simulink model "hexa_CAD_FxTDiff_ANSFT"  (R2023a)
settings: Solver=ode4  StartTime=0.0  StopTime=60  FixedStep=0.01  RelTol=1e-3
model workspace (MAT data in the model file):
  hover_2m = [0 0 2 0 0 0 0 0 2 0 0 0 ... (36 elements, 6x6)]
  square = [0 0 2.5 0 0 0 0 0 2.5 0 0 0 ... (36 elements, 6x6)]
  tf : Simulink.Parameter (value not decoded)
  tray0 = [0 0 0 0 0 0 0 0 5 0 0 0 ... (36 elements, 6x6)]
  tray1 = [0 0 0 0 0 0 0 0 5 0 0 0 ... (36 elements, 6x6)]
  tray2 = [0 0 0 0 0 0 2 0 5 0 0 0 ... (36 elements, 6x6)]
  tray3 = [0 0 0 0 0 0 2 0 5 0 0 0 ... (36 elements, 6x6)]
  tray4 = [0 0 0 0 0 0 2 0 5 0.15 0 0 ... (36 elements, 6x6)]
  tray5 = [0 0 0 0 0 0 0 0 5 0.15 0 0 ... (36 elements, 6x6)]
  tray_roll = [0 0 0 0.15 0 0 0 0 0 0.15 0 0 ... (36 elements, 6x6)]
  tray_yaw = [0 0 0 0 0 0 0 0 5 0 0 0 ... (36 elements, 6x6)]
undefined symbols (not defined in the file or in its folder): F, Light, MIL, smiData, X, Y, Z
libraries: sm_lib x230, nesl_utility x28, dspsrcs4 x6, simulink x3, sharedtransform x2, robotcorelib x1, aerolibwind2 x1, SignalEditorBlockLib x1
(part 6 of 6)

== system hexa_CAD_FxTDiff_ANSFT/6DoF_Dynamics/Hexa_Simsape/Raspberry_Pi_4_Model_B_STEP_1_RIGID/x2X_USB2_0_PORTS_RPi4ModelB_STEP_1_RIGID ==
  ReferenceFrame : sm_lib/Frames and Transforms/Reference Frame
  Solid : sm_lib/Body Elements/File Solid  ExtGeomFileName=2X USB2.0 PORTS- RPi4ModelB.STEP_Predeterminado_sldprt.STEP  UnitType=FromFile  ExtGeomFileUnits=m  StepReaderType=HEX  ExportConvexHullGeometry=off  InertiaType=Custom  Mass=smiData.Solid(25).mass  MassUnits=kg  CenterOfMass=smiData.Solid(25).CoM  CenterOfMassUnits=mm  MomentsOfInertia=smiData.Solid(25).MoI  MomentsOfInertiaUnits=kg*mm^2  ProductsOfInertia=smiData.Solid(25).PoI  ProductsOfInertiaUnits=kg*mm^2  BasedOnType=DensityFromFile  Density=1000  DensityUnits=kg/m^3  DoExposeReferenceFrame=on  SerializedFrames=<Frames/>  GraphicType=FromGeometry  MarkerShape=Sphere  MarkerSize=10  GraphicVisPropType=SimpleVisualProperties  GraphicDiffuseColor=smiData.Solid(25).color  GraphicSpecularColor=[0.5 0.5 0.5 1.0]  GraphicAmbientColor=[0.15 0.15 0.15 1.0]  GraphicEmissiveColor=[0.0 0.0 0.0 1.0]  GraphicShininess=75  GraphicOpacity=smiData.Solid(25).opacity
  F : PMIOPort  Side=Left
  connections:
  Solid/RConn1 -- ReferenceFrame/RConn1 -- F/RConn1

== system hexa_CAD_FxTDiff_ANSFT/6DoF_Dynamics/Hexa_Simsape/Raspberry_Pi_4_Model_B_STEP_1_RIGID/x2X_USB3_0_PORTS_RPi4ModelB_STEP_1_RIGID ==
  ReferenceFrame : sm_lib/Frames and Transforms/Reference Frame
  Solid : sm_lib/Body Elements/File Solid  ExtGeomFileName=2X USB3.0 PORTS- RPi4ModelB.STEP_Predeterminado_sldprt.STEP  UnitType=FromFile  ExtGeomFileUnits=m  StepReaderType=HEX  ExportConvexHullGeometry=off  InertiaType=Custom  Mass=smiData.Solid(11).mass  MassUnits=kg  CenterOfMass=smiData.Solid(11).CoM  CenterOfMassUnits=mm  MomentsOfInertia=smiData.Solid(11).MoI  MomentsOfInertiaUnits=kg*mm^2  ProductsOfInertia=smiData.Solid(11).PoI  ProductsOfInertiaUnits=kg*mm^2  BasedOnType=DensityFromFile  Density=1000  DensityUnits=kg/m^3  DoExposeReferenceFrame=on  SerializedFrames=<Frames/>  GraphicType=FromGeometry  MarkerShape=Sphere  MarkerSize=10  GraphicVisPropType=SimpleVisualProperties  GraphicDiffuseColor=smiData.Solid(11).color  GraphicSpecularColor=[0.5 0.5 0.5 1.0]  GraphicAmbientColor=[0.15 0.15 0.15 1.0]  GraphicEmissiveColor=[0.0 0.0 0.0 1.0]  GraphicShininess=75  GraphicOpacity=smiData.Solid(11).opacity
  F : PMIOPort  Side=Left
  connections:
  Solid/RConn1 -- ReferenceFrame/RConn1 -- F/RConn1

== system hexa_CAD_FxTDiff_ANSFT/6DoF_Dynamics/Hexa_Simsape/Raspberry_Pi_4_Model_B_STEP_1_RIGID/x2_54_mm_DUPONT_MALE_PIN_HEADER_IO_2X20_RPi4ModelB_STEP_1_RIGID ==
  ReferenceFrame : sm_lib/Frames and Transforms/Reference Frame
  Solid : sm_lib/Body Elements/File Solid  ExtGeomFileName=2.54 mm DUPONT MALE PIN HEADER- IO- 2X20- RPi4ModelB.STEP_Predeterminado_sldprt.STEP  UnitType=FromFile  ExtGeomFileUnits=m  StepReaderType=HEX  ExportConvexHullGeometry=off  InertiaType=Custom  Mass=smiData.Solid(21).mass  MassUnits=kg  CenterOfMass=smiData.Solid(21).CoM  CenterOfMassUnits=mm  MomentsOfInertia=smiData.Solid(21).MoI  MomentsOfInertiaUnits=kg*mm^2  ProductsOfInertia=smiData.Solid(21).PoI  ProductsOfInertiaUnits=kg*mm^2  BasedOnType=DensityFromFile  Density=1000  DensityUnits=kg/m^3  DoExposeReferenceFrame=on  SerializedFrames=<Frames/>  GraphicType=FromGeometry  MarkerShape=Sphere  MarkerSize=10  GraphicVisPropType=SimpleVisualProperties  GraphicDiffuseColor=smiData.Solid(21).color  GraphicSpecularColor=[0.5 0.5 0.5 1.0]  GraphicAmbientColor=[0.15 0.15 0.15 1.0]  GraphicEmissiveColor=[0.0 0.0 0.0 1.0]  GraphicShininess=75  GraphicOpacity=smiData.Solid(21).opacity
  F : PMIOPort  Side=Left
  connections:
  Solid/RConn1 -- ReferenceFrame/RConn1 -- F/RConn1

== system hexa_CAD_FxTDiff_ANSFT/6DoF_Dynamics/Hexa_Simsape/Raspberry_Pi_4_Model_B_STEP_1_RIGID/x2_54_mm_DUPONT_MALE_PIN_HEADER_POE_2X2_RPi4ModelB_STEP_1_RIGID ==
  ReferenceFrame : sm_lib/Frames and Transforms/Reference Frame
  Solid : sm_lib/Body Elements/File Solid  ExtGeomFileName=2.54 mm DUPONT MALE PIN HEADER- POE- 2X2- RPi4ModelB.STEP_Predeterminado_sldprt.STEP  UnitType=FromFile  ExtGeomFileUnits=m  StepReaderType=HEX  ExportConvexHullGeometry=off  InertiaType=Custom  Mass=smiData.Solid(20).mass  MassUnits=kg  CenterOfMass=smiData.Solid(20).CoM  CenterOfMassUnits=mm  MomentsOfInertia=smiData.Solid(20).MoI  MomentsOfInertiaUnits=kg*mm^2  ProductsOfInertia=smiData.Solid(20).PoI  ProductsOfInertiaUnits=kg*mm^2  BasedOnType=DensityFromFile  Density=1000  DensityUnits=kg/m^3  DoExposeReferenceFrame=on  SerializedFrames=<Frames/>  GraphicType=FromGeometry  MarkerShape=Sphere  MarkerSize=10  GraphicVisPropType=SimpleVisualProperties  GraphicDiffuseColor=smiData.Solid(20).color  GraphicSpecularColor=[0.5 0.5 0.5 1.0]  GraphicAmbientColor=[0.15 0.15 0.15 1.0]  GraphicEmissiveColor=[0.0 0.0 0.0 1.0]  GraphicShininess=75  GraphicOpacity=smiData.Solid(20).opacity
  F : PMIOPort  Side=Left
  connections:
  Solid/RConn1 -- ReferenceFrame/RConn1 -- F/RConn1

== system hexa_CAD_FxTDiff_ANSFT/6DoF_Dynamics/Hexa_Simsape/Raspberry_Pi_4_Model_B_STEP_1_RIGID/x91D77_D9WHV_778K_4_GB_LPDDR4_SDRAM_RPi4ModelB_STEP_1_RIGID ==
  ReferenceFrame : sm_lib/Frames and Transforms/Reference Frame
  Solid : sm_lib/Body Elements/File Solid  ExtGeomFileName=91D77 D9WHV 778K- 4 GB LPDDR4 SDRAM- RPi4ModelB.STEP_Predeterminado_sldprt.STEP  UnitType=FromFile  ExtGeomFileUnits=m  StepReaderType=HEX  ExportConvexHullGeometry=off  InertiaType=Custom  Mass=smiData.Solid(13).mass  MassUnits=kg  CenterOfMass=smiData.Solid(13).CoM  CenterOfMassUnits=mm  MomentsOfInertia=smiData.Solid(13).MoI  MomentsOfInertiaUnits=kg*mm^2  ProductsOfInertia=smiData.Solid(13).PoI  ProductsOfInertiaUnits=kg*mm^2  BasedOnType=DensityFromFile  Density=1000  DensityUnits=kg/m^3  DoExposeReferenceFrame=on  SerializedFrames=<Frames/>  GraphicType=FromGeometry  MarkerShape=Sphere  MarkerSize=10  GraphicVisPropType=SimpleVisualProperties  GraphicDiffuseColor=smiData.Solid(13).color  GraphicSpecularColor=[0.5 0.5 0.5 1.0]  GraphicAmbientColor=[0.15 0.15 0.15 1.0]  GraphicEmissiveColor=[0.0 0.0 0.0 1.0]  GraphicShininess=75  GraphicOpacity=smiData.Solid(13).opacity
  F : PMIOPort  Side=Left
  connections:
  Solid/RConn1 -- ReferenceFrame/RConn1 -- F/RConn1

== matlab function hexa_CAD_FxTDiff_ANSFT/Trajectory/Helicoidal Trajectory ==
  data: time input; pose_d output; pose_d_dot output; pose_d_ddot output
function [pose_d, pose_d_dot, pose_d_ddot]= fcn(time)

% pos_z = time / 12;
f = 0.15;
arg = f * (time - 5);
r = 2;

% hover for 5 s | include inclination in roll
% 5 metros al menos

if (time < 5)
    pos_x = 0;
    pos_y = 0;
    roll = 0;
    pos_z = 0.4 * time;
    yaw = 0;
else
    pos_x = -r + r * cos (arg);
    pos_y = r * sin (arg);
    pos_z = 2;
    roll = 0.15;
    yaw = (time - 5) * 2 * pi / 180; 
end

% roll = 0;
% yaw = time * 0;

pose_d = [pos_x;
          pos_y;
          pos_z;
          roll;
          0;
          yaw*0];

% pos_z_dot = 1 / 12;

% hover for 5 s
if (time < 5)
    pos_x_dot = 0;
    pos_y_dot = 0;
    pos_z_dot = 0.4;
    yaw_dot = 0;
else
    pos_x_dot = - f * r * sin(arg);
    pos_y_dot = f * r * cos(arg);
    pos_z_dot = 0;
    yaw_dot = 2 * pi / 180;
end

% yaw_dot = 0;

pose_d_dot = [pos_x_dot;
              pos_y_dot;
              pos_z_dot;
              0;
              0;
              yaw_dot*0];

pos_z_ddot = 0;
% hover for 5 s
if (time < 5)
    pos_x_ddot = 0;
    pos_y_ddot = 0;
else
    pos_x_ddot = - f * f * r * cos(arg);
    pos_y_ddot = - f * f * r * sin(arg);
end

pose_d_ddot = [pos_x_ddot;
               pos_y_ddot;
               pos_z_ddot;
               0;
               0;
               0];

== matlab function hexa_CAD_FxTDiff_ANSFT/Controller/ansftConstants ==
  data: xi1 output; xi2 output; lambda1 output; lambda2 output; alpha output; beta output; unused input
function [xi1, xi2, lambda1, lambda2, alpha, beta] = fcn(~)

%% Constantes de la Superficie deslizante
% zeta1 parecido a una ganancia proporcional
xi1 = [2.5; 2.5; 1.5; 1; 1; 1];
%zeta2 parecido a una ganancia derivatida
xi2 = [0.8; 0.8; 0.75; 0.5; 0.5; 0.5];
% lambda 1 > lambda2
lambda1 = [1.5; 1.5; 1.5; 2; 2; 2];
% 1 < lambda2 < 2
lambda2 = [1.33; 1.33; 1.25; 1.2; 1.2; 1.2];

%% Constantes del control auxiliar
%minimize sigma
alpha = [1.75; 1.75; 2; 3.75; 3.75; 1.25];

%aumetnar control, aumentar energía del sistema
beta = [2; 2; 1; 0.1; 0.1; 0.1];

== matlab function hexa_CAD_FxTDiff_ANSFT/Controller/calculateMassMatrix ==
  data: M output; M_inv output
function [M, M_inv] = fcn
m = 1.8;
Jxx = 0.11;
Jyy = 0.11;
Jzz = 0.0593;


M = [m, 0, 0, 0, 0, 0;
    0, m, 0, 0, 0, 0;
    0, 0, m, 0, 0, 0;
    0, 0, 0, Jxx, 0, 0;
    0, 0, 0, 0, Jyy, 0;
    0, 0, 0, 0, 0, Jzz];

M_inv = inv(M);

%% Fg matrix calculation

== matlab function hexa_CAD_FxTDiff_ANSFT/Trajectory/Lemniscate Trajectory ==
  data: time input; pose_d output; pose_d_dot output; pose_d_ddot output
function [pose_d, pose_d_dot, pose_d_ddot]= fcn(time)

%% Positions

arg = time / 4;

pos_x = cos(arg) ./ (1 + sin(arg) .* sin(arg));
pos_y = cos(arg) .* sin(arg) ./ (1 + sin(arg) .* sin(arg));
pos_z = time / 12;

yaw = time * 0;

pose_d = [pos_x;
          pos_y;
          pos_z;
          0;
          0;
          yaw];

%% Velocities

pos_z_dot = 1 / 12;
pos_x_dot = 0;
pos_y_dot = 0;
yaw_dot = 0;

pose_d_dot = [pos_x_dot;
              pos_y_dot;
              pos_z_dot;
              0;
              0;
              yaw_dot];

%% Accelerations

pos_z_ddot = 0;
pos_x_ddot = 0;
pos_y_ddot = 0;
yaw_ddot = 0;

pose_d_ddot = [pos_x_ddot;
               pos_y_ddot;
               pos_z_ddot;
               0;
               0;
               yaw_ddot];

== matlab function hexa_CAD_FxTDiff_ANSFT/Controller/calculatePWM ==
  data: omega2 input; pwm output
function pwm = fcn(omega2)

pwm = -1.3121e-09 .* omega2 .* omega2 + 0.00208 .* omega2 + 1107.922;

== matlab function hexa_CAD_FxTDiff_ANSFT/Controller/calculateActuationMatrix ==
  data: pose input; B output
function B  = fcn(pose)

roll = pose(4);
pitch = pose(5);
yaw = pose(6);

R1 = [cos(yaw)*cos(pitch), -cos(roll)*sin(yaw) + cos(yaw)*sin(roll)*sin(pitch), sin(roll)*sin(yaw) + cos(roll)*cos(yaw)*sin(pitch);
       cos(pitch)*sin(yaw), cos(roll)*cos(yaw) + sin(yaw)*sin(pitch)*sin(roll), -cos(yaw)*sin(roll) + sin(yaw)*sin(pitch)*cos(roll);
       -sin(pitch), cos(pitch)*sin(roll), cos(pitch)*cos(roll)];

R2 = [1, sin(roll)*tan(pitch), cos(roll)*tan(pitch);
      0, cos(roll), -sin(roll);
      0, sin(roll)/cos(pitch), cos(roll)/cos(pitch)];

Rzeros = zeros(3);

B = [transpose(R1), Rzeros;
     Rzeros, inv(R2)];

== matlab function hexa_CAD_FxTDiff_ANSFT/Fixed-Time Differentiator/ft_diff_gains ==
  data: G1 output; Q1 output; G2 output; Q2 output; lam1 output; lam2 output; vrho1 output; vrho2 output
function [G1, Q1, G2, Q2, lam1, lam2, vrho1, vrho2] = fcn

G1 = [5; 5; 5; 5; 5; 5];
Q1 = G1;
% 3 4 1.6
G2 = [6; 6; 6; 6; 6; 6];
Q2 = G2;

% mayor lam1, neor sensibilidad al ruido pero menor velocidad de
% convergencia
lam1 = [0.68, 0.68, 0.64, 0.64, 0.64, 0.64]';
vrho1 = [1.2, 1.2, 1.2, 1.2, 1.2, 1.2]';
lam2 = 2 * lam1 - 1;
vrho2 = 2 * vrho1 - 1;

== matlab function hexa_CAD_FxTDiff_ANSFT/Controller/calculatePhiMatrix ==
  data: Phi output; v input
function Phi  = fcn(v)

%% Phi matrix calculation
uu = v(1);
vv = v(2);
ww = v(3);
pp = v(4);
qq = v(5);
rr = v(6);


Phi = [0, -rr, qq, 0, -ww, vv;
        rr, 0, -pp , ww, 0, -uu;
        -qq, pp, 0,  -vv, uu, 0;
        0, 0, 0, 0, -rr, qq; 
        0, 0, 0, rr, 0, -pp;
        0, 0, 0, -qq, pp, 0];

Phi = transpose(Phi);

== matlab function hexa_CAD_FxTDiff_ANSFT/Controller/calculateRotationMatrix ==
  data: pose input; Rbi output
function Rbi  = fcn(pose)

roll = pose(4);
pitch = pose(5);
yaw = pose(6);

R1 = [cos(yaw)*cos(pitch), -cos(roll)*sin(yaw) + cos(yaw)*sin(roll)*sin(pitch), sin(roll)*sin(yaw) + cos(roll)*cos(yaw)*sin(pitch);
       cos(pitch)*sin(yaw), cos(roll)*cos(yaw) + sin(yaw)*sin(pitch)*sin(roll), -cos(yaw)*sin(roll) + sin(yaw)*sin(pitch)*cos(roll);
       -sin(pitch), cos(pitch)*sin(roll), cos(pitch)*cos(roll)];

R2 = [1, sin(roll)*tan(pitch), cos(roll)*tan(pitch);
      0, cos(roll), -sin(roll);
      0, sin(roll)/cos(pitch), cos(roll)/cos(pitch)];

Rzeros = zeros(3);

Rbi = [transpose(R1), Rzeros;
       Rzeros, inv(R2)];
